simulink model "suspension_simulink"  (R2025b)
settings: Solver=ode45  StartTime=0.0  StopTime=10.0  RelTol=1e-3
settings Model: Creator=raul  LastModifiedBy=raul

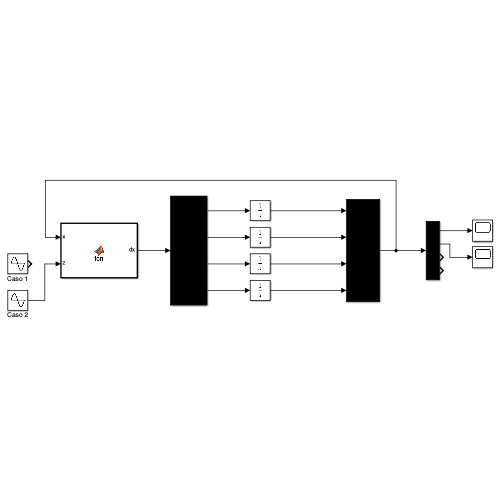
[thumbnail: Simulink's stored preview of the top-level diagram]
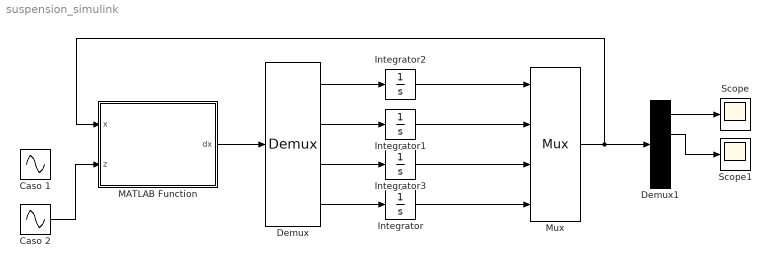
== system suspension_simulink ==
  Caso 1 : Sin  Amplitude=0.05  Frequency=0.5*pi  SampleTime=0
  Caso 2 : Sin  Amplitude=0.05  Frequency=20*pi  SampleTime=0
  Demux : Demux
  Demux1 : Demux
  Integrator{,1..3} (4 alike) : Integrator
  MATLAB Function : MATLAB Function  TreatAsAtomicUnit=on
  Mux : Mux
  Scope : Scope
      settings: ActiveDisplayYMinimum=-0.0044757265597088081  ActiveDisplayYMaximum=0.0055408205366274032
  Scope1 : Scope
      settings: ActiveDisplayYMinimum=-0.0081004107203282542  ActiveDisplayYMaximum=0.013153550265285606
  wires:
  Demux/4 -> Integrator/1
  MATLAB Function/1(dx) -> Demux/1
  Demux/1 -> Integrator2/1
  Demux/2 -> Integrator1/1
  Demux/3 -> Integrator3/1
  Integrator/1 -> Mux/4
  Integrator3/1 -> Mux/3
  Integrator1/1 -> Mux/2
  Integrator2/1 -> Mux/1
  Mux/1 -> Demux1/1, MATLAB Function/1(x)
  Demux1/1 -> Scope/1
  Demux1/2 -> Scope1/1
  Caso 2/1 -> MATLAB Function/2(z)

== matlab function suspension_simulink/MATLAB Function ==
  data: x input; dx output; z input
function dx = fcn(x, z)

m1 = 290;
m2 = 59;
b1 = 1000;
k1 = 16182;
k2 = 19000;
f  = 0;

dx = zeros(4,1);

dx(1) = x(3);
dx(2) = x(4);

dx(3) = (-b1*(x(3) - x(4)) - k1*(x(1) - x(2)) + f) / m1;

dx(4) = (b1*(x(3) - x(4)) + k1*(x(1) - x(2)) - k2*(x(2) - z) - f) / m2;
